simulink model "autoCreatedModel"  (R2023a)
settings: Solver=FixedStepDiscrete  StartTime=0.0  StopTime=10.0  FixedStep=0.1  RelTol=1e-3
undefined symbols (not defined in the file or in its folder): Batt_AncOutVoltage, Batt_BalancingRequired, Batt_BMSStatus, Batt_BoostChargeActive, Batt_ChargeContactorStatus, Batt_ClearFault_Code, Batt_ClearFault_KeyMatched, Batt_Coolant_IN_Pressure, Batt_Coolant_IN_Temp, Batt_Coolant_OUT_Pressure, Batt_Coolant_OUT_Temp, Batt_Current, Batt_DischargePowerLim, Batt_DischargePowerLim_2s, Batt_DischargePowerLim_5s, Batt_DischEnergyThroughput, Batt_EnergyAvailable, Batt_Equity_SoC_Displayed, Batt_Fault_FR0, Batt_Fault_FR1, Batt_Fault_FR2, Batt_Fault_FR3, Batt_Fault_FR4, Batt_Fault_FR5, Batt_Fault_FR6, Batt_Fault_FR7, Batt_FaultActive_FR4, Batt_HVILFault, Batt_InvOutVoltage, Batt_Isolation1OnOffStatus, Batt_Isolation1Res_HighRange, Batt_Isolation1Resistance, Batt_Isolation1Status, Batt_Isolation2OnOffStatus, Batt_Isolation2Status, Batt_LoggerPercent, Batt_LVBackupBattVoltage, Batt_LVVoltage, Batt_MainContactorStatus, Batt_MaxCellTemperature, Batt_MaxCellVoltage, Batt_MaxSOC, Batt_MinCellTemperature, Batt_MinCellVoltage, Batt_MinSOC, Batt_ReadyforBoostCharge, Batt_ReadytoTurnOnHV, Batt_RegenPowerLim, Batt_RegenPowerLim_2s, Batt_RegenPowerLim_5s, Batt_SafetyLightStatGreenHV, Batt_SafetyLightStatRedHV, Batt_SerialNumber, Batt_ThermalRequest, Batt_UserSOC, Batt_Voltage, BMS, BMS_AliveCounter1, BMS_AliveCounter2, BMS_AliveCounter3 ... (+154)
libraries: canoelib x133
(part 1 of 2)
settings Model: Creator=DIL  LastModifiedBy=DIL

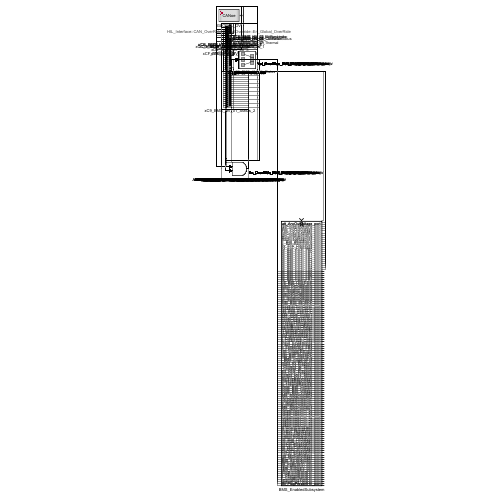
[thumbnail: Simulink's stored preview of the top-level diagram]
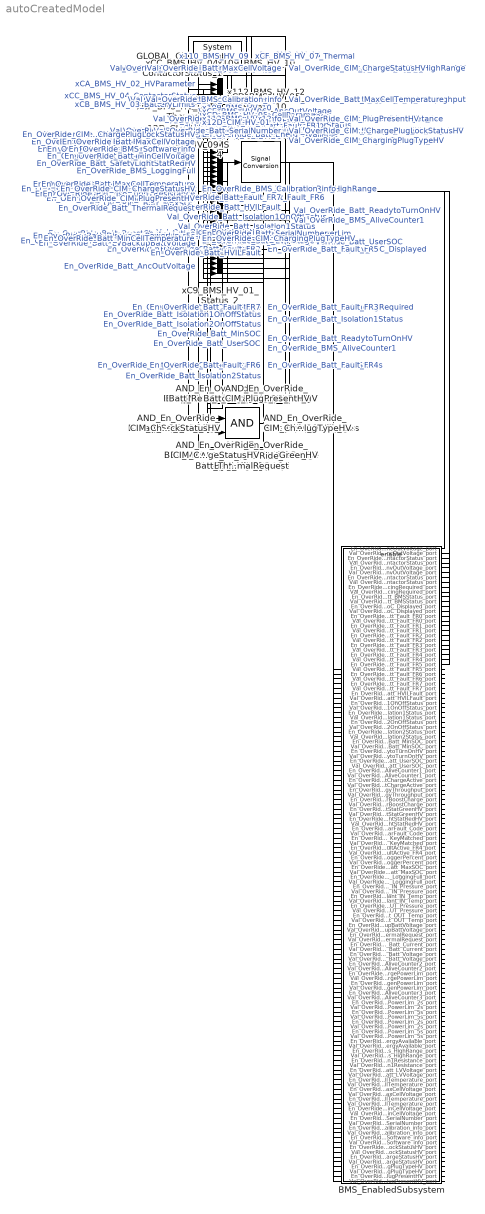
== system autoCreatedModel ==
  AND_En_OverRide_BMS_AliveCounter1 : Logic  IconShape=distinctive  AllPortsSameDT=off  OutDataTypeStr=boolean
  AND_En_OverRide_BMS_AliveCounter2 : Logic  IconShape=distinctive  AllPortsSameDT=off  OutDataTypeStr=boolean
  AND_En_OverRide_BMS_AliveCounter3 : Logic  IconShape=distinctive  AllPortsSameDT=off  OutDataTypeStr=boolean
  AND_En_OverRide_BMS_Calibration_info : Logic  IconShape=distinctive  AllPortsSameDT=off  OutDataTypeStr=boolean
  AND_En_OverRide_BMS_LoggingFull : Logic  IconShape=distinctive  AllPortsSameDT=off  OutDataTypeStr=boolean
  AND_En_OverRide_BMS_Software_info : Logic  IconShape=distinctive  AllPortsSameDT=off  OutDataTypeStr=boolean
  AND_En_OverRide_Batt_AncOutVoltage : Logic  IconShape=distinctive  AllPortsSameDT=off  OutDataTypeStr=boolean
  AND_En_OverRide_Batt_BMSStatus : Logic  IconShape=distinctive  AllPortsSameDT=off  OutDataTypeStr=boolean
  AND_En_OverRide_Batt_BalancingRequired : Logic  IconShape=distinctive  AllPortsSameDT=off  OutDataTypeStr=boolean
  AND_En_OverRide_Batt_BoostChargeActive : Logic  IconShape=distinctive  AllPortsSameDT=off  OutDataTypeStr=boolean
  AND_En_OverRide_Batt_ChargeContactorStatus : Logic  IconShape=distinctive  AllPortsSameDT=off  OutDataTypeStr=boolean
  AND_En_OverRide_Batt_ClearFault_Code : Logic  IconShape=distinctive  AllPortsSameDT=off  OutDataTypeStr=boolean
  AND_En_OverRide_Batt_ClearFault_KeyMatched : Logic  IconShape=distinctive  AllPortsSameDT=off  OutDataTypeStr=boolean
  AND_En_OverRide_Batt_Coolant_IN_Pressure : Logic  IconShape=distinctive  AllPortsSameDT=off  OutDataTypeStr=boolean
  AND_En_OverRide_Batt_Coolant_IN_Temp : Logic  IconShape=distinctive  AllPortsSameDT=off  OutDataTypeStr=boolean
  AND_En_OverRide_Batt_Coolant_OUT_Pressure : Logic  IconShape=distinctive  AllPortsSameDT=off  OutDataTypeStr=boolean
  AND_En_OverRide_Batt_Coolant_OUT_Temp : Logic  IconShape=distinctive  AllPortsSameDT=off  OutDataTypeStr=boolean
  AND_En_OverRide_Batt_Current : Logic  IconShape=distinctive  AllPortsSameDT=off  OutDataTypeStr=boolean
  AND_En_OverRide_Batt_DischEnergyThroughput : Logic  IconShape=distinctive  AllPortsSameDT=off  OutDataTypeStr=boolean
  AND_En_OverRide_Batt_DischargePowerLim : Logic  IconShape=distinctive  AllPortsSameDT=off  OutDataTypeStr=boolean
  AND_En_OverRide_Batt_DischargePowerLim_2s : Logic  IconShape=distinctive  AllPortsSameDT=off  OutDataTypeStr=boolean
  AND_En_OverRide_Batt_DischargePowerLim_5s : Logic  IconShape=distinctive  AllPortsSameDT=off  OutDataTypeStr=boolean
  AND_En_OverRide_Batt_EnergyAvailable : Logic  IconShape=distinctive  AllPortsSameDT=off  OutDataTypeStr=boolean
  AND_En_OverRide_Batt_Equity_SoC_Displayed : Logic  IconShape=distinctive  AllPortsSameDT=off  OutDataTypeStr=boolean
  AND_En_OverRide_Batt_FaultActive_FR4 : Logic  IconShape=distinctive  AllPortsSameDT=off  OutDataTypeStr=boolean
  AND_En_OverRide_Batt_Fault_FR{0..7} (8 alike) : Logic  IconShape=distinctive  AllPortsSameDT=off  OutDataTypeStr=boolean
  AND_En_OverRide_Batt_HVILFault : Logic  IconShape=distinctive  AllPortsSameDT=off  OutDataTypeStr=boolean
  AND_En_OverRide_Batt_InvOutVoltage : Logic  IconShape=distinctive  AllPortsSameDT=off  OutDataTypeStr=boolean
  AND_En_OverRide_Batt_Isolation1OnOffStatus : Logic  IconShape=distinctive  AllPortsSameDT=off  OutDataTypeStr=boolean
  AND_En_OverRide_Batt_Isolation1Res_HighRange : Logic  IconShape=distinctive  AllPortsSameDT=off  OutDataTypeStr=boolean
  AND_En_OverRide_Batt_Isolation1Resistance : Logic  IconShape=distinctive  AllPortsSameDT=off  OutDataTypeStr=boolean
  AND_En_OverRide_Batt_Isolation1Status : Logic  IconShape=distinctive  AllPortsSameDT=off  OutDataTypeStr=boolean
  AND_En_OverRide_Batt_Isolation2OnOffStatus : Logic  IconShape=distinctive  AllPortsSameDT=off  OutDataTypeStr=boolean
  AND_En_OverRide_Batt_Isolation2Status : Logic  IconShape=distinctive  AllPortsSameDT=off  OutDataTypeStr=boolean
  AND_En_OverRide_Batt_LVBackupBattVoltage : Logic  IconShape=distinctive  AllPortsSameDT=off  OutDataTypeStr=boolean
  AND_En_OverRide_Batt_LVVoltage : Logic  IconShape=distinctive  AllPortsSameDT=off  OutDataTypeStr=boolean
  AND_En_OverRide_Batt_LoggerPercent : Logic  IconShape=distinctive  AllPortsSameDT=off  OutDataTypeStr=boolean
  AND_En_OverRide_Batt_MainContactorStatus : Logic  IconShape=distinctive  AllPortsSameDT=off  OutDataTypeStr=boolean
  AND_En_OverRide_Batt_MaxCellTemperature : Logic  IconShape=distinctive  AllPortsSameDT=off  OutDataTypeStr=boolean
  AND_En_OverRide_Batt_MaxCellVoltage : Logic  IconShape=distinctive  AllPortsSameDT=off  OutDataTypeStr=boolean
  AND_En_OverRide_Batt_MaxSOC : Logic  IconShape=distinctive  AllPortsSameDT=off  OutDataTypeStr=boolean
  AND_En_OverRide_Batt_MinCellTemperature : Logic  IconShape=distinctive  AllPortsSameDT=off  OutDataTypeStr=boolean
  AND_En_OverRide_Batt_MinCellVoltage : Logic  IconShape=distinctive  AllPortsSameDT=off  OutDataTypeStr=boolean
  AND_En_OverRide_Batt_MinSOC : Logic  IconShape=distinctive  AllPortsSameDT=off  OutDataTypeStr=boolean
  AND_En_OverRide_Batt_ReadyforBoostCharge : Logic  IconShape=distinctive  AllPortsSameDT=off  OutDataTypeStr=boolean
  AND_En_OverRide_Batt_ReadytoTurnOnHV : Logic  IconShape=distinctive  AllPortsSameDT=off  OutDataTypeStr=boolean
  AND_En_OverRide_Batt_RegenPowerLim : Logic  IconShape=distinctive  AllPortsSameDT=off  OutDataTypeStr=boolean
  AND_En_OverRide_Batt_RegenPowerLim_2s : Logic  IconShape=distinctive  AllPortsSameDT=off  OutDataTypeStr=boolean
  AND_En_OverRide_Batt_RegenPowerLim_5s : Logic  IconShape=distinctive  AllPortsSameDT=off  OutDataTypeStr=boolean
  AND_En_OverRide_Batt_SafetyLightStatGreenHV : Logic  IconShape=distinctive  AllPortsSameDT=off  OutDataTypeStr=boolean
  AND_En_OverRide_Batt_SafetyLightStatRedHV : Logic  IconShape=distinctive  AllPortsSameDT=off  OutDataTypeStr=boolean
  AND_En_OverRide_Batt_SerialNumber : Logic  IconShape=distinctive  AllPortsSameDT=off  OutDataTypeStr=boolean
  AND_En_OverRide_Batt_ThermalRequest : Logic  IconShape=distinctive  AllPortsSameDT=off  OutDataTypeStr=boolean
  AND_En_OverRide_Batt_UserSOC : Logic  IconShape=distinctive  AllPortsSameDT=off  OutDataTypeStr=boolean
  AND_En_OverRide_Batt_Voltage : Logic  IconShape=distinctive  AllPortsSameDT=off  OutDataTypeStr=boolean
  AND_En_OverRide_CIM_ChargePlugLockStatusHV : Logic  IconShape=distinctive  AllPortsSameDT=off  OutDataTypeStr=boolean
  AND_En_OverRide_CIM_ChargeStatusHV : Logic  IconShape=distinctive  AllPortsSameDT=off  OutDataTypeStr=boolean
  AND_En_OverRide_CIM_ChargingPlugTypeHV : Logic  IconShape=distinctive  AllPortsSameDT=off  OutDataTypeStr=boolean
  AND_En_OverRide_CIM_PlugPresentHV : Logic  IconShape=distinctive  AllPortsSameDT=off  OutDataTypeStr=boolean
  BMS : BusCreator  Inputs=12
  BMS_EnabledSubsystem : Subsystem  TreatAsAtomicUnit=on
  GLOBAL_OV : canoelib/CANoe I//O/System Variable Input  nsName=HIL_Interface  sysVarName=CAN_OverRide::GlobalOverride::En_Global_OverRide  arrayIndex=-1  editSampleTime=0.001  rawValue=Default  dataType=Default  dataTypeDB=unknown  hasEncoding=off  dataTypeCANoe=Get from CANoe
      settings: AttributesFormatString=%<nsName>::%<sysVarName>  SourceProductName=Vector CANoe
  SignalConvertion{1..132} (132 alike) : SignalConversion  OverrideOpt=off
  x109_BMS_HV_10_8 : BusCreator  Inputs=8
  x110_BMS_HV_09_4 : BusCreator  Inputs=12
  x112_BMS_HV_12_11 : BusCreator  Inputs=6
  x12D_CIM_HV_01_12 : BusCreator  Inputs=8
  xC9_BMS_HV_01_Status_2 : BusCreator  Inputs=40
  xCA_BMS_HV_02_HVParameter_6 : BusCreator  Inputs=6
  xCB_BMS_HV_03_BatteryLimits_7 : BusCreator  Inputs=6
  xCC_BMS_HV_04_ContactorStatus_1 : BusCreator  Inputs=8
  xCD_BMS_HV_05_CellParam_10 : BusCreator  Inputs=8
  xCE_BMS_HV_06_9 : BusCreator  Inputs=8
  xCF_BMS_HV_07_Thermal_5 : BusCreator  Inputs=12
  xD2_BMS_HV_08_3 : BusCreator  Inputs=10
  wires:
  BMS_EnabledSubsystem/1(En_OverRide_Batt_AncOutVoltage_port) -> SignalConvertion1/1
  GLOBAL_OV/1 -> AND_En_OverRide_Batt_AncOutVoltage/1, AND_En_OverRide_Batt_ChargeContactorStatus/1, AND_En_OverRide_Batt_InvOutVoltage/1, AND_En_OverRide_Batt_MainContactorStatus/1, AND_En_OverRide_Batt_BalancingRequired/1, AND_En_OverRide_Batt_BMSStatus/1, AND_En_OverRide_Batt_Equity_SoC_Displayed/1, AND_En_OverRide_Batt_Fault_FR0/1, AND_En_OverRide_Batt_Fault_FR1/1, AND_En_OverRide_Batt_Fault_FR2/1, AND_En_OverRide_Batt_Fault_FR3/1, AND_En_OverRide_Batt_Fault_FR4/1, AND_En_OverRide_Batt_Fault_FR5/1, AND_En_OverRide_Batt_Fault_FR6/1, AND_En_OverRide_Batt_Fault_FR7/1, AND_En_OverRide_Batt_HVILFault/1, AND_En_OverRide_Batt_Isolation1OnOffStatus/1, AND_En_OverRide_Batt_Isolation1Status/1, AND_En_OverRide_Batt_Isolation2OnOffStatus/1, AND_En_OverRide_Batt_Isolation2Status/1, AND_En_OverRide_Batt_MinSOC/1, AND_En_OverRide_Batt_ReadytoTurnOnHV/1, AND_En_OverRide_Batt_UserSOC/1, AND_En_OverRide_BMS_AliveCounter1/1, AND_En_OverRide_Batt_BoostChargeActive/1, AND_En_OverRide_Batt_DischEnergyThroughput/1, AND_En_OverRide_Batt_ReadyforBoostCharge/1, AND_En_OverRide_Batt_SafetyLightStatGreenHV/1, AND_En_OverRide_Batt_SafetyLightStatRedHV/1, AND_En_OverRide_Batt_ClearFault_Code/1, AND_En_OverRide_Batt_ClearFault_KeyMatched/1, AND_En_OverRide_Batt_FaultActive_FR4/1, AND_En_OverRide_Batt_LoggerPercent/1, AND_En_OverRide_Batt_MaxSOC/1, AND_En_OverRide_BMS_LoggingFull/1, AND_En_OverRide_Batt_Coolant_IN_Pressure/1, AND_En_OverRide_Batt_Coolant_IN_Temp/1, AND_En_OverRide_Batt_Coolant_OUT_Pressure/1, AND_En_OverRide_Batt_Coolant_OUT_Temp/1, AND_En_OverRide_Batt_LVBackupBattVoltage/1, AND_En_OverRide_Batt_ThermalRequest/1, AND_En_OverRide_Batt_Current/1, AND_En_OverRide_Batt_Voltage/1, AND_En_OverRide_BMS_AliveCounter2/1, AND_En_OverRide_Batt_DischargePowerLim/1, AND_En_OverRide_Batt_RegenPowerLim/1, AND_En_OverRide_BMS_AliveCounter3/1, AND_En_OverRide_Batt_DischargePowerLim_2s/1, AND_En_OverRide_Batt_DischargePowerLim_5s/1, AND_En_OverRide_Batt_RegenPowerLim_2s/1, AND_En_OverRide_Batt_RegenPowerLim_5s/1, AND_En_OverRide_Batt_EnergyAvailable/1, AND_En_OverRide_Batt_Isolation1Res_HighRange/1, AND_En_OverRide_Batt_Isolation1Resistance/1, AND_En_OverRide_Batt_LVVoltage/1, AND_En_OverRide_Batt_MaxCellTemperature/1, AND_En_OverRide_Batt_MaxCellVoltage/1, AND_En_OverRide_Batt_MinCellTemperature/1, AND_En_OverRide_Batt_MinCellVoltage/1, AND_En_OverRide_Batt_SerialNumber/1, AND_En_OverRide_BMS_Calibration_info/1, AND_En_OverRide_BMS_Software_info/1, AND_En_OverRide_CIM_ChargePlugLockStatusHV/1, AND_En_OverRide_CIM_ChargeStatusHV/1, AND_En_OverRide_CIM_ChargingPlugTypeHV/1, AND_En_OverRide_CIM_PlugPresentHV/1
  SignalConvertion1/1 -> AND_En_OverRide_Batt_AncOutVoltage/2
  AND_En_OverRide_Batt_AncOutVoltage/1 -> xCC_BMS_HV_04_ContactorStatus_1/1  "En_OverRide_Batt_AncOutVoltage"
  BMS_EnabledSubsystem/2(Val_OverRide_Batt_AncOutVoltage_port) -> SignalConvertion2/1
  SignalConvertion2/1 -> xCC_BMS_HV_04_ContactorStatus_1/2  "Val_OverRide_Batt_AncOutVoltage"
  BMS_EnabledSubsystem/3(En_OverRide_Batt_ChargeContactorStatus_port) -> SignalConvertion3/1
  SignalConvertion3/1 -> AND_En_OverRide_Batt_ChargeContactorStatus/2
  AND_En_OverRide_Batt_ChargeContactorStatus/1 -> xCC_BMS_HV_04_ContactorStatus_1/3  "En_OverRide_Batt_ChargeContactorStatus"
  BMS_EnabledSubsystem/4(Val_OverRide_Batt_ChargeContactorStatus_port) -> SignalConvertion4/1
  SignalConvertion4/1 -> xCC_BMS_HV_04_ContactorStatus_1/4  "Val_OverRide_Batt_ChargeContactorStatus"
  BMS_EnabledSubsystem/5(En_OverRide_Batt_InvOutVoltage_port) -> SignalConvertion5/1
  SignalConvertion5/1 -> AND_En_OverRide_Batt_InvOutVoltage/2
  AND_En_OverRide_Batt_InvOutVoltage/1 -> xCC_BMS_HV_04_ContactorStatus_1/5  "En_OverRide_Batt_InvOutVoltage"
  BMS_EnabledSubsystem/6(Val_OverRide_Batt_InvOutVoltage_port) -> SignalConvertion6/1
  SignalConvertion6/1 -> xCC_BMS_HV_04_ContactorStatus_1/6  "Val_OverRide_Batt_InvOutVoltage"
  BMS_EnabledSubsystem/7(En_OverRide_Batt_MainContactorStatus_port) -> SignalConvertion7/1
  SignalConvertion7/1 -> AND_En_OverRide_Batt_MainContactorStatus/2
  AND_En_OverRide_Batt_MainContactorStatus/1 -> xCC_BMS_HV_04_ContactorStatus_1/7  "En_OverRide_Batt_MainContactorStatus"
  BMS_EnabledSubsystem/8(Val_OverRide_Batt_MainContactorStatus_port) -> SignalConvertion8/1
  SignalConvertion8/1 -> xCC_BMS_HV_04_ContactorStatus_1/8  "Val_OverRide_Batt_MainContactorStatus"
  xCC_BMS_HV_04_ContactorStatus_1/1 -> BMS/1  "xCC_BMS_HV_04_ContactorStatus"
  BMS_EnabledSubsystem/9(En_OverRide_Batt_BalancingRequired_port) -> SignalConvertion9/1
  SignalConvertion9/1 -> AND_En_OverRide_Batt_BalancingRequired/2
  AND_En_OverRide_Batt_BalancingRequired/1 -> xC9_BMS_HV_01_Status_2/1  "En_OverRide_Batt_BalancingRequired"
  BMS_EnabledSubsystem/10(Val_OverRide_Batt_BalancingRequired_port) -> SignalConvertion10/1
  SignalConvertion10/1 -> xC9_BMS_HV_01_Status_2/2  "Val_OverRide_Batt_BalancingRequired"
  BMS_EnabledSubsystem/11(En_OverRide_Batt_BMSStatus_port) -> SignalConvertion11/1
  SignalConvertion11/1 -> AND_En_OverRide_Batt_BMSStatus/2
  AND_En_OverRide_Batt_BMSStatus/1 -> xC9_BMS_HV_01_Status_2/3  "En_OverRide_Batt_BMSStatus"
  BMS_EnabledSubsystem/12(Val_OverRide_Batt_BMSStatus_port) -> SignalConvertion12/1
  SignalConvertion12/1 -> xC9_BMS_HV_01_Status_2/4  "Val_OverRide_Batt_BMSStatus"
  BMS_EnabledSubsystem/13(En_OverRide_Batt_Equity_SoC_Displayed_port) -> SignalConvertion13/1
  SignalConvertion13/1 -> AND_En_OverRide_Batt_Equity_SoC_Displayed/2
  AND_En_OverRide_Batt_Equity_SoC_Displayed/1 -> xC9_BMS_HV_01_Status_2/5  "En_OverRide_Batt_Equity_SoC_Displayed"
  BMS_EnabledSubsystem/14(Val_OverRide_Batt_Equity_SoC_Displayed_port) -> SignalConvertion14/1
  SignalConvertion14/1 -> xC9_BMS_HV_01_Status_2/6  "Val_OverRide_Batt_Equity_SoC_Displayed"
  BMS_EnabledSubsystem/15(En_OverRide_Batt_Fault_FR0_port) -> SignalConvertion15/1
  SignalConvertion15/1 -> AND_En_OverRide_Batt_Fault_FR0/2
  AND_En_OverRide_Batt_Fault_FR0/1 -> xC9_BMS_HV_01_Status_2/7  "En_OverRide_Batt_Fault_FR0"
  BMS_EnabledSubsystem/16(Val_OverRide_Batt_Fault_FR0_port) -> SignalConvertion16/1
  SignalConvertion16/1 -> xC9_BMS_HV_01_Status_2/8  "Val_OverRide_Batt_Fault_FR0"
  BMS_EnabledSubsystem/17(En_OverRide_Batt_Fault_FR1_port) -> SignalConvertion17/1
  SignalConvertion17/1 -> AND_En_OverRide_Batt_Fault_FR1/2
  AND_En_OverRide_Batt_Fault_FR1/1 -> xC9_BMS_HV_01_Status_2/9  "En_OverRide_Batt_Fault_FR1"
  BMS_EnabledSubsystem/18(Val_OverRide_Batt_Fault_FR1_port) -> SignalConvertion18/1
  SignalConvertion18/1 -> xC9_BMS_HV_01_Status_2/10  "Val_OverRide_Batt_Fault_FR1"
  BMS_EnabledSubsystem/19(En_OverRide_Batt_Fault_FR2_port) -> SignalConvertion19/1
  SignalConvertion19/1 -> AND_En_OverRide_Batt_Fault_FR2/2
  AND_En_OverRide_Batt_Fault_FR2/1 -> xC9_BMS_HV_01_Status_2/11  "En_OverRide_Batt_Fault_FR2"
  BMS_EnabledSubsystem/20(Val_OverRide_Batt_Fault_FR2_port) -> SignalConvertion20/1
  SignalConvertion20/1 -> xC9_BMS_HV_01_Status_2/12  "Val_OverRide_Batt_Fault_FR2"
  BMS_EnabledSubsystem/21(En_OverRide_Batt_Fault_FR3_port) -> SignalConvertion21/1
  SignalConvertion21/1 -> AND_En_OverRide_Batt_Fault_FR3/2
  AND_En_OverRide_Batt_Fault_FR3/1 -> xC9_BMS_HV_01_Status_2/13  "En_OverRide_Batt_Fault_FR3"
  BMS_EnabledSubsystem/22(Val_OverRide_Batt_Fault_FR3_port) -> SignalConvertion22/1
  SignalConvertion22/1 -> xC9_BMS_HV_01_Status_2/14  "Val_OverRide_Batt_Fault_FR3"
  BMS_EnabledSubsystem/23(En_OverRide_Batt_Fault_FR4_port) -> SignalConvertion23/1
  SignalConvertion23/1 -> AND_En_OverRide_Batt_Fault_FR4/2
  AND_En_OverRide_Batt_Fault_FR4/1 -> xC9_BMS_HV_01_Status_2/15  "En_OverRide_Batt_Fault_FR4"
  BMS_EnabledSubsystem/24(Val_OverRide_Batt_Fault_FR4_port) -> SignalConvertion24/1
  SignalConvertion24/1 -> xC9_BMS_HV_01_Status_2/16  "Val_OverRide_Batt_Fault_FR4"
  BMS_EnabledSubsystem/25(En_OverRide_Batt_Fault_FR5_port) -> SignalConvertion25/1
  SignalConvertion25/1 -> AND_En_OverRide_Batt_Fault_FR5/2
  AND_En_OverRide_Batt_Fault_FR5/1 -> xC9_BMS_HV_01_Status_2/17  "En_OverRide_Batt_Fault_FR5"
  BMS_EnabledSubsystem/26(Val_OverRide_Batt_Fault_FR5_port) -> SignalConvertion26/1
  SignalConvertion26/1 -> xC9_BMS_HV_01_Status_2/18  "Val_OverRide_Batt_Fault_FR5"
  BMS_EnabledSubsystem/27(En_OverRide_Batt_Fault_FR6_port) -> SignalConvertion27/1
  SignalConvertion27/1 -> AND_En_OverRide_Batt_Fault_FR6/2
  AND_En_OverRide_Batt_Fault_FR6/1 -> xC9_BMS_HV_01_Status_2/19  "En_OverRide_Batt_Fault_FR6"
  BMS_EnabledSubsystem/28(Val_OverRide_Batt_Fault_FR6_port) -> SignalConvertion28/1
  SignalConvertion28/1 -> xC9_BMS_HV_01_Status_2/20  "Val_OverRide_Batt_Fault_FR6"
  BMS_EnabledSubsystem/29(En_OverRide_Batt_Fault_FR7_port) -> SignalConvertion29/1
  SignalConvertion29/1 -> AND_En_OverRide_Batt_Fault_FR7/2
  AND_En_OverRide_Batt_Fault_FR7/1 -> xC9_BMS_HV_01_Status_2/21  "En_OverRide_Batt_Fault_FR7"
  BMS_EnabledSubsystem/30(Val_OverRide_Batt_Fault_FR7_port) -> SignalConvertion30/1
  SignalConvertion30/1 -> xC9_BMS_HV_01_Status_2/22  "Val_OverRide_Batt_Fault_FR7"
  BMS_EnabledSubsystem/31(En_OverRide_Batt_HVILFault_port) -> SignalConvertion31/1
  SignalConvertion31/1 -> AND_En_OverRide_Batt_HVILFault/2
  AND_En_OverRide_Batt_HVILFault/1 -> xC9_BMS_HV_01_Status_2/23  "En_OverRide_Batt_HVILFault"
  BMS_EnabledSubsystem/32(Val_OverRide_Batt_HVILFault_port) -> SignalConvertion32/1
  SignalConvertion32/1 -> xC9_BMS_HV_01_Status_2/24  "Val_OverRide_Batt_HVILFault"
  BMS_EnabledSubsystem/33(En_OverRide_Batt_Isolation1OnOffStatus_port) -> SignalConvertion33/1
  SignalConvertion33/1 -> AND_En_OverRide_Batt_Isolation1OnOffStatus/2
  AND_En_OverRide_Batt_Isolation1OnOffStatus/1 -> xC9_BMS_HV_01_Status_2/25  "En_OverRide_Batt_Isolation1OnOffStatus"
  BMS_EnabledSubsystem/34(Val_OverRide_Batt_Isolation1OnOffStatus_port) -> SignalConvertion34/1
  SignalConvertion34/1 -> xC9_BMS_HV_01_Status_2/26  "Val_OverRide_Batt_Isolation1OnOffStatus"
  BMS_EnabledSubsystem/35(En_OverRide_Batt_Isolation1Status_port) -> SignalConvertion35/1
  SignalConvertion35/1 -> AND_En_OverRide_Batt_Isolation1Status/2
  AND_En_OverRide_Batt_Isolation1Status/1 -> xC9_BMS_HV_01_Status_2/27  "En_OverRide_Batt_Isolation1Status"
  BMS_EnabledSubsystem/36(Val_OverRide_Batt_Isolation1Status_port) -> SignalConvertion36/1
  SignalConvertion36/1 -> xC9_BMS_HV_01_Status_2/28  "Val_OverRide_Batt_Isolation1Status"
  BMS_EnabledSubsystem/37(En_OverRide_Batt_Isolation2OnOffStatus_port) -> SignalConvertion37/1
  SignalConvertion37/1 -> AND_En_OverRide_Batt_Isolation2OnOffStatus/2
  AND_En_OverRide_Batt_Isolation2OnOffStatus/1 -> xC9_BMS_HV_01_Status_2/29  "En_OverRide_Batt_Isolation2OnOffStatus"
  BMS_EnabledSubsystem/38(Val_OverRide_Batt_Isolation2OnOffStatus_port) -> SignalConvertion38/1
  SignalConvertion38/1 -> xC9_BMS_HV_01_Status_2/30  "Val_OverRide_Batt_Isolation2OnOffStatus"
  BMS_EnabledSubsystem/39(En_OverRide_Batt_Isolation2Status_port) -> SignalConvertion39/1
  SignalConvertion39/1 -> AND_En_OverRide_Batt_Isolation2Status/2
  AND_En_OverRide_Batt_Isolation2Status/1 -> xC9_BMS_HV_01_Status_2/31  "En_OverRide_Batt_Isolation2Status"
  BMS_EnabledSubsystem/40(Val_OverRide_Batt_Isolation2Status_port) -> SignalConvertion40/1
  SignalConvertion40/1 -> xC9_BMS_HV_01_Status_2/32  "Val_OverRide_Batt_Isolation2Status"
  BMS_EnabledSubsystem/41(En_OverRide_Batt_MinSOC_port) -> SignalConvertion41/1
  SignalConvertion41/1 -> AND_En_OverRide_Batt_MinSOC/2
  AND_En_OverRide_Batt_MinSOC/1 -> xC9_BMS_HV_01_Status_2/33  "En_OverRide_Batt_MinSOC"
  BMS_EnabledSubsystem/42(Val_OverRide_Batt_MinSOC_port) -> SignalConvertion42/1
  SignalConvertion42/1 -> xC9_BMS_HV_01_Status_2/34  "Val_OverRide_Batt_MinSOC"
  BMS_EnabledSubsystem/43(En_OverRide_Batt_ReadytoTurnOnHV_port) -> SignalConvertion43/1
  SignalConvertion43/1 -> AND_En_OverRide_Batt_ReadytoTurnOnHV/2
  AND_En_OverRide_Batt_ReadytoTurnOnHV/1 -> xC9_BMS_HV_01_Status_2/35  "En_OverRide_Batt_ReadytoTurnOnHV"
  BMS_EnabledSubsystem/44(Val_OverRide_Batt_ReadytoTurnOnHV_port) -> SignalConvertion44/1
  SignalConvertion44/1 -> xC9_BMS_HV_01_Status_2/36  "Val_OverRide_Batt_ReadytoTurnOnHV"
  BMS_EnabledSubsystem/45(En_OverRide_Batt_UserSOC_port) -> SignalConvertion45/1
  SignalConvertion45/1 -> AND_En_OverRide_Batt_UserSOC/2
  AND_En_OverRide_Batt_UserSOC/1 -> xC9_BMS_HV_01_Status_2/37  "En_OverRide_Batt_UserSOC"
  BMS_EnabledSubsystem/46(Val_OverRide_Batt_UserSOC_port) -> SignalConvertion46/1
  SignalConvertion46/1 -> xC9_BMS_HV_01_Status_2/38  "Val_OverRide_Batt_UserSOC"
  BMS_EnabledSubsystem/47(En_OverRide_BMS_AliveCounter1_port) -> SignalConvertion47/1
  SignalConvertion47/1 -> AND_En_OverRide_BMS_AliveCounter1/2
  AND_En_OverRide_BMS_AliveCounter1/1 -> xC9_BMS_HV_01_Status_2/39  "En_OverRide_BMS_AliveCounter1"
  BMS_EnabledSubsystem/48(Val_OverRide_BMS_AliveCounter1_port) -> SignalConvertion48/1
  SignalConvertion48/1 -> xC9_BMS_HV_01_Status_2/40  "Val_OverRide_BMS_AliveCounter1"
  xC9_BMS_HV_01_Status_2/1 -> BMS/2  "xC9_BMS_HV_01_Status"
  BMS_EnabledSubsystem/49(En_OverRide_Batt_BoostChargeActive_port) -> SignalConvertion49/1
  SignalConvertion49/1 -> AND_En_OverRide_Batt_BoostChargeActive/2
  AND_En_OverRide_Batt_BoostChargeActive/1 -> xD2_BMS_HV_08_3/1  "En_OverRide_Batt_BoostChargeActive"
  BMS_EnabledSubsystem/50(Val_OverRide_Batt_BoostChargeActive_port) -> SignalConvertion50/1
  SignalConvertion50/1 -> xD2_BMS_HV_08_3/2  "Val_OverRide_Batt_BoostChargeActive"
  BMS_EnabledSubsystem/51(En_OverRide_Batt_DischEnergyThroughput_port) -> SignalConvertion51/1
  SignalConvertion51/1 -> AND_En_OverRide_Batt_DischEnergyThroughput/2
  AND_En_OverRide_Batt_DischEnergyThroughput/1 -> xD2_BMS_HV_08_3/3  "En_OverRide_Batt_DischEnergyThroughput"
  BMS_EnabledSubsystem/52(Val_OverRide_Batt_DischEnergyThroughput_port) -> SignalConvertion52/1
  SignalConvertion52/1 -> xD2_BMS_HV_08_3/4  "Val_OverRide_Batt_DischEnergyThroughput"
  BMS_EnabledSubsystem/53(En_OverRide_Batt_ReadyforBoostCharge_port) -> SignalConvertion53/1
  SignalConvertion53/1 -> AND_En_OverRide_Batt_ReadyforBoostCharge/2
  AND_En_OverRide_Batt_ReadyforBoostCharge/1 -> xD2_BMS_HV_08_3/5  "En_OverRide_Batt_ReadyforBoostCharge"
  BMS_EnabledSubsystem/54(Val_OverRide_Batt_ReadyforBoostCharge_port) -> SignalConvertion54/1
  SignalConvertion54/1 -> xD2_BMS_HV_08_3/6  "Val_OverRide_Batt_ReadyforBoostCharge"
  BMS_EnabledSubsystem/55(En_OverRide_Batt_SafetyLightStatGreenHV_port) -> SignalConvertion55/1
  SignalConvertion55/1 -> AND_En_OverRide_Batt_SafetyLightStatGreenHV/2
  AND_En_OverRide_Batt_SafetyLightStatGreenHV/1 -> xD2_BMS_HV_08_3/7  "En_OverRide_Batt_SafetyLightStatGreenHV"
  BMS_EnabledSubsystem/56(Val_OverRide_Batt_SafetyLightStatGreenHV_port) -> SignalConvertion56/1
  SignalConvertion56/1 -> xD2_BMS_HV_08_3/8  "Val_OverRide_Batt_SafetyLightStatGreenHV"
  BMS_EnabledSubsystem/57(En_OverRide_Batt_SafetyLightStatRedHV_port) -> SignalConvertion57/1
  SignalConvertion57/1 -> AND_En_OverRide_Batt_SafetyLightStatRedHV/2
  AND_En_OverRide_Batt_SafetyLightStatRedHV/1 -> xD2_BMS_HV_08_3/9  "En_OverRide_Batt_SafetyLightStatRedHV"
  BMS_EnabledSubsystem/58(Val_OverRide_Batt_SafetyLightStatRedHV_port) -> SignalConvertion58/1
  SignalConvertion58/1 -> xD2_BMS_HV_08_3/10  "Val_OverRide_Batt_SafetyLightStatRedHV"
  xD2_BMS_HV_08_3/1 -> BMS/3  "xD2_BMS_HV_08"
  BMS_EnabledSubsystem/59(En_OverRide_Batt_ClearFault_Code_port) -> SignalConvertion59/1
  SignalConvertion59/1 -> AND_En_OverRide_Batt_ClearFault_Code/2
  AND_En_OverRide_Batt_ClearFault_Code/1 -> x110_BMS_HV_09_4/1  "En_OverRide_Batt_ClearFault_Code"
  BMS_EnabledSubsystem/60(Val_OverRide_Batt_ClearFault_Code_port) -> SignalConvertion60/1
  SignalConvertion60/1 -> x110_BMS_HV_09_4/2  "Val_OverRide_Batt_ClearFault_Code"
  BMS_EnabledSubsystem/61(En_OverRide_Batt_ClearFault_KeyMatched_port) -> SignalConvertion61/1
  SignalConvertion61/1 -> AND_En_OverRide_Batt_ClearFault_KeyMatched/2
  AND_En_OverRide_Batt_ClearFault_KeyMatched/1 -> x110_BMS_HV_09_4/3  "En_OverRide_Batt_ClearFault_KeyMatched"
  BMS_EnabledSubsystem/62(Val_OverRide_Batt_ClearFault_KeyMatched_port) -> SignalConvertion62/1
  SignalConvertion62/1 -> x110_BMS_HV_09_4/4  "Val_OverRide_Batt_ClearFault_KeyMatched"
  BMS_EnabledSubsystem/63(En_OverRide_Batt_FaultActive_FR4_port) -> SignalConvertion63/1
  SignalConvertion63/1 -> AND_En_OverRide_Batt_FaultActive_FR4/2
  AND_En_OverRide_Batt_FaultActive_FR4/1 -> x110_BMS_HV_09_4/5  "En_OverRide_Batt_FaultActive_FR4"
  BMS_EnabledSubsystem/64(Val_OverRide_Batt_FaultActive_FR4_port) -> SignalConvertion64/1
  SignalConvertion64/1 -> x110_BMS_HV_09_4/6  "Val_OverRide_Batt_FaultActive_FR4"
  BMS_EnabledSubsystem/65(En_OverRide_Batt_LoggerPercent_port) -> SignalConvertion65/1
  SignalConvertion65/1 -> AND_En_OverRide_Batt_LoggerPercent/2
  AND_En_OverRide_Batt_LoggerPercent/1 -> x110_BMS_HV_09_4/7  "En_OverRide_Batt_LoggerPercent"
  BMS_EnabledSubsystem/66(Val_OverRide_Batt_LoggerPercent_port) -> SignalConvertion66/1
  SignalConvertion66/1 -> x110_BMS_HV_09_4/8  "Val_OverRide_Batt_LoggerPercent"
  BMS_EnabledSubsystem/67(En_OverRide_Batt_MaxSOC_port) -> SignalConvertion67/1
  SignalConvertion67/1 -> AND_En_OverRide_Batt_MaxSOC/2
  AND_En_OverRide_Batt_MaxSOC/1 -> x110_BMS_HV_09_4/9  "En_OverRide_Batt_MaxSOC"
  BMS_EnabledSubsystem/68(Val_OverRide_Batt_MaxSOC_port) -> SignalConvertion68/1
  SignalConvertion68/1 -> x110_BMS_HV_09_4/10  "Val_OverRide_Batt_MaxSOC"
  BMS_EnabledSubsystem/69(En_OverRide_BMS_LoggingFull_port) -> SignalConvertion69/1
  SignalConvertion69/1 -> AND_En_OverRide_BMS_LoggingFull/2
  AND_En_OverRide_BMS_LoggingFull/1 -> x110_BMS_HV_09_4/11  "En_OverRide_BMS_LoggingFull"
  BMS_EnabledSubsystem/70(Val_OverRide_BMS_LoggingFull_port) -> SignalConvertion70/1
  SignalConvertion70/1 -> x110_BMS_HV_09_4/12  "Val_OverRide_BMS_LoggingFull"
  x110_BMS_HV_09_4/1 -> BMS/4  "x110_BMS_HV_09"
  BMS_EnabledSubsystem/71(En_OverRide_Batt_Coolant_IN_Pressure_port) -> SignalConvertion71/1
  SignalConvertion71/1 -> AND_En_OverRide_Batt_Coolant_IN_Pressure/2
  AND_En_OverRide_Batt_Coolant_IN_Pressure/1 -> xCF_BMS_HV_07_Thermal_5/1  "En_OverRide_Batt_Coolant_IN_Pressure"
  BMS_EnabledSubsystem/72(Val_OverRide_Batt_Coolant_IN_Pressure_port) -> SignalConvertion72/1
  SignalConvertion72/1 -> xCF_BMS_HV_07_Thermal_5/2  "Val_OverRide_Batt_Coolant_IN_Pressure"
  BMS_EnabledSubsystem/73(En_OverRide_Batt_Coolant_IN_Temp_port) -> SignalConvertion73/1
  SignalConvertion73/1 -> AND_En_OverRide_Batt_Coolant_IN_Temp/2
  AND_En_OverRide_Batt_Coolant_IN_Temp/1 -> xCF_BMS_HV_07_Thermal_5/3  "En_OverRide_Batt_Coolant_IN_Temp"
  BMS_EnabledSubsystem/74(Val_OverRide_Batt_Coolant_IN_Temp_port) -> SignalConvertion74/1
  SignalConvertion74/1 -> xCF_BMS_HV_07_Thermal_5/4  "Val_OverRide_Batt_Coolant_IN_Temp"
  BMS_EnabledSubsystem/75(En_OverRide_Batt_Coolant_OUT_Pressure_port) -> SignalConvertion75/1
  SignalConvertion75/1 -> AND_En_OverRide_Batt_Coolant_OUT_Pressure/2
  AND_En_OverRide_Batt_Coolant_OUT_Pressure/1 -> xCF_BMS_HV_07_Thermal_5/5  "En_OverRide_Batt_Coolant_OUT_Pressure"
  BMS_EnabledSubsystem/76(Val_OverRide_Batt_Coolant_OUT_Pressure_port) -> SignalConvertion76/1
  SignalConvertion76/1 -> xCF_BMS_HV_07_Thermal_5/6  "Val_OverRide_Batt_Coolant_OUT_Pressure"
  BMS_EnabledSubsystem/77(En_OverRide_Batt_Coolant_OUT_Temp_port) -> SignalConvertion77/1
  SignalConvertion77/1 -> AND_En_OverRide_Batt_Coolant_OUT_Temp/2
  AND_En_OverRide_Batt_Coolant_OUT_Temp/1 -> xCF_BMS_HV_07_Thermal_5/7  "En_OverRide_Batt_Coolant_OUT_Temp"
  BMS_EnabledSubsystem/78(Val_OverRide_Batt_Coolant_OUT_Temp_port) -> SignalConvertion78/1
  SignalConvertion78/1 -> xCF_BMS_HV_07_Thermal_5/8  "Val_OverRide_Batt_Coolant_OUT_Temp"
  BMS_EnabledSubsystem/79(En_OverRide_Batt_LVBackupBattVoltage_port) -> SignalConvertion79/1
  SignalConvertion79/1 -> AND_En_OverRide_Batt_LVBackupBattVoltage/2
  AND_En_OverRide_Batt_LVBackupBattVoltage/1 -> xCF_BMS_HV_07_Thermal_5/9  "En_OverRide_Batt_LVBackupBattVoltage"
  BMS_EnabledSubsystem/80(Val_OverRide_Batt_LVBackupBattVoltage_port) -> SignalConvertion80/1
  SignalConvertion80/1 -> xCF_BMS_HV_07_Thermal_5/10  "Val_OverRide_Batt_LVBackupBattVoltage"
  BMS_EnabledSubsystem/81(En_OverRide_Batt_ThermalRequest_port) -> SignalConvertion81/1
  SignalConvertion81/1 -> AND_En_OverRide_Batt_ThermalRequest/2
  AND_En_OverRide_Batt_ThermalRequest/1 -> xCF_BMS_HV_07_Thermal_5/11  "En_OverRide_Batt_ThermalRequest"
  BMS_EnabledSubsystem/82(Val_OverRide_Batt_ThermalRequest_port) -> SignalConvertion82/1
  SignalConvertion82/1 -> xCF_BMS_HV_07_Thermal_5/12  "Val_OverRide_Batt_ThermalRequest"
  xCF_BMS_HV_07_Thermal_5/1 -> BMS/5  "xCF_BMS_HV_07_Thermal"
  BMS_EnabledSubsystem/83(En_OverRide_Batt_Current_port) -> SignalConvertion83/1
  SignalConvertion83/1 -> AND_En_OverRide_Batt_Current/2
  AND_En_OverRide_Batt_Current/1 -> xCA_BMS_HV_02_HVParameter_6/1  "En_OverRide_Batt_Current"
  BMS_EnabledSubsystem/84(Val_OverRide_Batt_Current_port) -> SignalConvertion84/1
  SignalConvertion84/1 -> xCA_BMS_HV_02_HVParameter_6/2  "Val_OverRide_Batt_Current"
  BMS_EnabledSubsystem/85(En_OverRide_Batt_Voltage_port) -> SignalConvertion85/1
  SignalConvertion85/1 -> AND_En_OverRide_Batt_Voltage/2
  AND_En_OverRide_Batt_Voltage/1 -> xCA_BMS_HV_02_HVParameter_6/3  "En_OverRide_Batt_Voltage"
  BMS_EnabledSubsystem/86(Val_OverRide_Batt_Voltage_port) -> SignalConvertion86/1
  SignalConvertion86/1 -> xCA_BMS_HV_02_HVParameter_6/4  "Val_OverRide_Batt_Voltage"
  BMS_EnabledSubsystem/87(En_OverRide_BMS_AliveCounter2_port) -> SignalConvertion87/1
  SignalConvertion87/1 -> AND_En_OverRide_BMS_AliveCounter2/2
  AND_En_OverRide_BMS_AliveCounter2/1 -> xCA_BMS_HV_02_HVParameter_6/5  "En_OverRide_BMS_AliveCounter2"
  BMS_EnabledSubsystem/88(Val_OverRide_BMS_AliveCounter2_port) -> SignalConvertion88/1
  SignalConvertion88/1 -> xCA_BMS_HV_02_HVParameter_6/6  "Val_OverRide_BMS_AliveCounter2"
  xCA_BMS_HV_02_HVParameter_6/1 -> BMS/6  "xCA_BMS_HV_02_HVParameter"
  BMS_EnabledSubsystem/89(En_OverRide_Batt_DischargePowerLim_port) -> SignalConvertion89/1
  SignalConvertion89/1 -> AND_En_OverRide_Batt_DischargePowerLim/2
  AND_En_OverRide_Batt_DischargePowerLim/1 -> xCB_BMS_HV_03_BatteryLimits_7/1  "En_OverRide_Batt_DischargePowerLim"
  BMS_EnabledSubsystem/90(Val_OverRide_Batt_DischargePowerLim_port) -> SignalConvertion90/1
  SignalConvertion90/1 -> xCB_BMS_HV_03_BatteryLimits_7/2  "Val_OverRide_Batt_DischargePowerLim"
  BMS_EnabledSubsystem/91(En_OverRide_Batt_RegenPowerLim_port) -> SignalConvertion91/1
  SignalConvertion91/1 -> AND_En_OverRide_Batt_RegenPowerLim/2
  AND_En_OverRide_Batt_RegenPowerLim/1 -> xCB_BMS_HV_03_BatteryLimits_7/3  "En_OverRide_Batt_RegenPowerLim"
  BMS_EnabledSubsystem/92(Val_OverRide_Batt_RegenPowerLim_port) -> SignalConvertion92/1
  SignalConvertion92/1 -> xCB_BMS_HV_03_BatteryLimits_7/4  "Val_OverRide_Batt_RegenPowerLim"
  BMS_EnabledSubsystem/93(En_OverRide_BMS_AliveCounter3_port) -> SignalConvertion93/1
  SignalConvertion93/1 -> AND_En_OverRide_BMS_AliveCounter3/2
  AND_En_OverRide_BMS_AliveCounter3/1 -> xCB_BMS_HV_03_BatteryLimits_7/5  "En_OverRide_BMS_AliveCounter3"
  BMS_EnabledSubsystem/94(Val_OverRide_BMS_AliveCounter3_port) -> SignalConvertion94/1
  SignalConvertion94/1 -> xCB_BMS_HV_03_BatteryLimits_7/6  "Val_OverRide_BMS_AliveCounter3"
  xCB_BMS_HV_03_BatteryLimits_7/1 -> BMS/7  "xCB_BMS_HV_03_BatteryLimits"
  BMS_EnabledSubsystem/95(En_OverRide_Batt_DischargePowerLim_2s_port) -> SignalConvertion95/1
  SignalConvertion95/1 -> AND_En_OverRide_Batt_DischargePowerLim_2s/2
  AND_En_OverRide_Batt_DischargePowerLim_2s/1 -> x109_BMS_HV_10_8/1  "En_OverRide_Batt_DischargePowerLim_2s"
  BMS_EnabledSubsystem/96(Val_OverRide_Batt_DischargePowerLim_2s_port) -> SignalConvertion96/1
  SignalConvertion96/1 -> x109_BMS_HV_10_8/2  "Val_OverRide_Batt_DischargePowerLim_2s"
  BMS_EnabledSubsystem/97(En_OverRide_Batt_DischargePowerLim_5s_port) -> SignalConvertion97/1
  SignalConvertion97/1 -> AND_En_OverRide_Batt_DischargePowerLim_5s/2
  AND_En_OverRide_Batt_DischargePowerLim_5s/1 -> x109_BMS_HV_10_8/3  "En_OverRide_Batt_DischargePowerLim_5s"
  BMS_EnabledSubsystem/98(Val_OverRide_Batt_DischargePowerLim_5s_port) -> SignalConvertion98/1
  SignalConvertion98/1 -> x109_BMS_HV_10_8/4  "Val_OverRide_Batt_DischargePowerLim_5s"
  BMS_EnabledSubsystem/99(En_OverRide_Batt_RegenPowerLim_2s_port) -> SignalConvertion99/1
  SignalConvertion99/1 -> AND_En_OverRide_Batt_RegenPowerLim_2s/2
  AND_En_OverRide_Batt_RegenPowerLim_2s/1 -> x109_BMS_HV_10_8/5  "En_OverRide_Batt_RegenPowerLim_2s"
  BMS_EnabledSubsystem/100(Val_OverRide_Batt_RegenPowerLim_2s_port) -> SignalConvertion100/1
  SignalConvertion100/1 -> x109_BMS_HV_10_8/6  "Val_OverRide_Batt_RegenPowerLim_2s"
  BMS_EnabledSubsystem/101(En_OverRide_Batt_RegenPowerLim_5s_port) -> SignalConvertion101/1
  SignalConvertion101/1 -> AND_En_OverRide_Batt_RegenPowerLim_5s/2
  AND_En_OverRide_Batt_RegenPowerLim_5s/1 -> x109_BMS_HV_10_8/7  "En_OverRide_Batt_RegenPowerLim_5s"
  BMS_EnabledSubsystem/102(Val_OverRide_Batt_RegenPowerLim_5s_port) -> SignalConvertion102/1
  SignalConvertion102/1 -> x109_BMS_HV_10_8/8  "Val_OverRide_Batt_RegenPowerLim_5s"
  x109_BMS_HV_10_8/1 -> BMS/8  "x109_BMS_HV_10"
  BMS_EnabledSubsystem/103(En_OverRide_Batt_EnergyAvailable_port) -> SignalConvertion103/1
  SignalConvertion103/1 -> AND_En_OverRide_Batt_EnergyAvailable/2
  AND_En_OverRide_Batt_EnergyAvailable/1 -> xCE_BMS_HV_06_9/1  "En_OverRide_Batt_EnergyAvailable"
  BMS_EnabledSubsystem/104(Val_OverRide_Batt_EnergyAvailable_port) -> SignalConvertion104/1
  SignalConvertion104/1 -> xCE_BMS_HV_06_9/2  "Val_OverRide_Batt_EnergyAvailable"
  BMS_EnabledSubsystem/105(En_OverRide_Batt_Isolation1Res_HighRange_port) -> SignalConvertion105/1
  SignalConvertion105/1 -> AND_En_OverRide_Batt_Isolation1Res_HighRange/2
  AND_En_OverRide_Batt_Isolation1Res_HighRange/1 -> xCE_BMS_HV_06_9/3  "En_OverRide_Batt_Isolation1Res_HighRange"
  BMS_EnabledSubsystem/106(Val_OverRide_Batt_Isolation1Res_HighRange_port) -> SignalConvertion106/1
  SignalConvertion106/1 -> xCE_BMS_HV_06_9/4  "Val_OverRide_Batt_Isolation1Res_HighRange"
  BMS_EnabledSubsystem/107(En_OverRide_Batt_Isolation1Resistance_port) -> SignalConvertion107/1
  SignalConvertion107/1 -> AND_En_OverRide_Batt_Isolation1Resistance/2
  AND_En_OverRide_Batt_Isolation1Resistance/1 -> xCE_BMS_HV_06_9/5  "En_OverRide_Batt_Isolation1Resistance"
  BMS_EnabledSubsystem/108(Val_OverRide_Batt_Isolation1Resistance_port) -> SignalConvertion108/1
  SignalConvertion108/1 -> xCE_BMS_HV_06_9/6  "Val_OverRide_Batt_Isolation1Resistance"
  BMS_EnabledSubsystem/109(En_OverRide_Batt_LVVoltage_port) -> SignalConvertion109/1
  SignalConvertion109/1 -> AND_En_OverRide_Batt_LVVoltage/2
  AND_En_OverRide_Batt_LVVoltage/1 -> xCE_BMS_HV_06_9/7  "En_OverRide_Batt_LVVoltage"
  BMS_EnabledSubsystem/110(Val_OverRide_Batt_LVVoltage_port) -> SignalConvertion110/1
  SignalConvertion110/1 -> xCE_BMS_HV_06_9/8  "Val_OverRide_Batt_LVVoltage"
  xCE_BMS_HV_06_9/1 -> BMS/9  "xCE_BMS_HV_06"
  BMS_EnabledSubsystem/111(En_OverRide_Batt_MaxCellTemperature_port) -> SignalConvertion111/1
  SignalConvertion111/1 -> AND_En_OverRide_Batt_MaxCellTemperature/2
  AND_En_OverRide_Batt_MaxCellTemperature/1 -> xCD_BMS_HV_05_CellParam_10/1  "En_OverRide_Batt_MaxCellTemperature"
  BMS_EnabledSubsystem/112(Val_OverRide_Batt_MaxCellTemperature_port) -> SignalConvertion112/1
  SignalConvertion112/1 -> xCD_BMS_HV_05_CellParam_10/2  "Val_OverRide_Batt_MaxCellTemperature"
  BMS_EnabledSubsystem/113(En_OverRide_Batt_MaxCellVoltage_port) -> SignalConvertion113/1
  SignalConvertion113/1 -> AND_En_OverRide_Batt_MaxCellVoltage/2
  AND_En_OverRide_Batt_MaxCellVoltage/1 -> xCD_BMS_HV_05_CellParam_10/3  "En_OverRide_Batt_MaxCellVoltage"
  BMS_EnabledSubsystem/114(Val_OverRide_Batt_MaxCellVoltage_port) -> SignalConvertion114/1
  SignalConvertion114/1 -> xCD_BMS_HV_05_CellParam_10/4  "Val_OverRide_Batt_MaxCellVoltage"
  BMS_EnabledSubsystem/115(En_OverRide_Batt_MinCellTemperature_port) -> SignalConvertion115/1
  SignalConvertion115/1 -> AND_En_OverRide_Batt_MinCellTemperature/2
  AND_En_OverRide_Batt_MinCellTemperature/1 -> xCD_BMS_HV_05_CellParam_10/5  "En_OverRide_Batt_MinCellTemperature"
  BMS_EnabledSubsystem/116(Val_OverRide_Batt_MinCellTemperature_port) -> SignalConvertion116/1
  SignalConvertion116/1 -> xCD_BMS_HV_05_CellParam_10/6  "Val_OverRide_Batt_MinCellTemperature"
  BMS_EnabledSubsystem/117(En_OverRide_Batt_MinCellVoltage_port) -> SignalConvertion117/1
  SignalConvertion117/1 -> AND_En_OverRide_Batt_MinCellVoltage/2
  AND_En_OverRide_Batt_MinCellVoltage/1 -> xCD_BMS_HV_05_CellParam_10/7  "En_OverRide_Batt_MinCellVoltage"
  BMS_EnabledSubsystem/118(Val_OverRide_Batt_MinCellVoltage_port) -> SignalConvertion118/1
  SignalConvertion118/1 -> xCD_BMS_HV_05_CellParam_10/8  "Val_OverRide_Batt_MinCellVoltage"
  xCD_BMS_HV_05_CellParam_10/1 -> BMS/10  "xCD_BMS_HV_05_CellParam"
  BMS_EnabledSubsystem/119(En_OverRide_Batt_SerialNumber_port) -> SignalConvertion119/1
  SignalConvertion119/1 -> AND_En_OverRide_Batt_SerialNumber/2
  AND_En_OverRide_Batt_SerialNumber/1 -> x112_BMS_HV_12_11/1  "En_OverRide_Batt_SerialNumber"
  BMS_EnabledSubsystem/120(Val_OverRide_Batt_SerialNumber_port) -> SignalConvertion120/1
  SignalConvertion120/1 -> x112_BMS_HV_12_11/2  "Val_OverRide_Batt_SerialNumber"
  BMS_EnabledSubsystem/121(En_OverRide_BMS_Calibration_info_port) -> SignalConvertion121/1
  SignalConvertion121/1 -> AND_En_OverRide_BMS_Calibration_info/2
  AND_En_OverRide_BMS_Calibration_info/1 -> x112_BMS_HV_12_11/3  "En_OverRide_BMS_Calibration_info"
  BMS_EnabledSubsystem/122(Val_OverRide_BMS_Calibration_info_port) -> SignalConvertion122/1
  SignalConvertion122/1 -> x112_BMS_HV_12_11/4  "Val_OverRide_BMS_Calibration_info"
  BMS_EnabledSubsystem/123(En_OverRide_BMS_Software_info_port) -> SignalConvertion123/1
  SignalConvertion123/1 -> AND_En_OverRide_BMS_Software_info/2
  AND_En_OverRide_BMS_Software_info/1 -> x112_BMS_HV_12_11/5  "En_OverRide_BMS_Software_info"
  BMS_EnabledSubsystem/124(Val_OverRide_BMS_Software_info_port) -> SignalConvertion124/1
  SignalConvertion124/1 -> x112_BMS_HV_12_11/6  "Val_OverRide_BMS_Software_info"
  x112_BMS_HV_12_11/1 -> BMS/11  "x112_BMS_HV_12"
  BMS_EnabledSubsystem/125(En_OverRide_CIM_ChargePlugLockStatusHV_port) -> SignalConvertion125/1
  SignalConvertion125/1 -> AND_En_OverRide_CIM_ChargePlugLockStatusHV/2
  AND_En_OverRide_CIM_ChargePlugLockStatusHV/1 -> x12D_CIM_HV_01_12/1  "En_OverRide_CIM_ChargePlugLockStatusHV"
  BMS_EnabledSubsystem/126(Val_OverRide_CIM_ChargePlugLockStatusHV_port) -> SignalConvertion126/1
  SignalConvertion126/1 -> x12D_CIM_HV_01_12/2  "Val_OverRide_CIM_ChargePlugLockStatusHV"
  BMS_EnabledSubsystem/127(En_OverRide_CIM_ChargeStatusHV_port) -> SignalConvertion127/1
  SignalConvertion127/1 -> AND_En_OverRide_CIM_ChargeStatusHV/2
  AND_En_OverRide_CIM_ChargeStatusHV/1 -> x12D_CIM_HV_01_12/3  "En_OverRide_CIM_ChargeStatusHV"
  BMS_EnabledSubsystem/128(Val_OverRide_CIM_ChargeStatusHV_port) -> SignalConvertion128/1
  SignalConvertion128/1 -> x12D_CIM_HV_01_12/4  "Val_OverRide_CIM_ChargeStatusHV"
  BMS_EnabledSubsystem/129(En_OverRide_CIM_ChargingPlugTypeHV_port) -> SignalConvertion129/1
  SignalConvertion129/1 -> AND_En_OverRide_CIM_ChargingPlugTypeHV/2
  AND_En_OverRide_CIM_ChargingPlugTypeHV/1 -> x12D_CIM_HV_01_12/5  "En_OverRide_CIM_ChargingPlugTypeHV"
  BMS_EnabledSubsystem/130(Val_OverRide_CIM_ChargingPlugTypeHV_port) -> SignalConvertion130/1
  SignalConvertion130/1 -> x12D_CIM_HV_01_12/6  "Val_OverRide_CIM_ChargingPlugTypeHV"
  BMS_EnabledSubsystem/131(En_OverRide_CIM_PlugPresentHV_port) -> SignalConvertion131/1
  SignalConvertion131/1 -> AND_En_OverRide_CIM_PlugPresentHV/2
  AND_En_OverRide_CIM_PlugPresentHV/1 -> x12D_CIM_HV_01_12/7  "En_OverRide_CIM_PlugPresentHV"
  BMS_EnabledSubsystem/132(Val_OverRide_CIM_PlugPresentHV_port) -> SignalConvertion132/1
  SignalConvertion132/1 -> x12D_CIM_HV_01_12/8  "Val_OverRide_CIM_PlugPresentHV"
  x12D_CIM_HV_01_12/1 -> BMS/12  "x12D_CIM_HV_01"
